simulink model "Copy_of_RL_Single_phase"  (R2020b)
settings: Solver=FixedStepDiscrete  StartTime=0.0  StopTime=Tfinal  FixedStep=SampleTime  RelTol=1e-3
InitFcn:
  | param
values from neighbouring files (symbols this model uses):
  C_DC = 1e-6    (= 1e-06)    [param.m]
  COUT = 100e-6    (= 0.0001)    [param.m]
  Cp = 1/(4*wr^2*Lp)    (= 3.29821561336e-08)    [param.m]
  Cs = 1/(4*wr^2*Ls)    (= 3.29821561336e-08)    [param.m]
  ESRA = 1e-7    (= 1e-07)    [param.m]
  ESRB = 1e-7    (= 1e-07)    [param.m]
  LCAHA = 1e-7    (= 1e-07)    [param.m]
  LCBHB = 1e-7    (= 1e-07)    [param.m]
  LHACB = 1e-7    (= 1e-07)    [param.m]
  LLoad = 2e-3    (= 0.002)    [param.m]
  Lp = 120e-6    (= 0.00012)    [param.m]
  Ls = 120e-6    (= 0.00012)    [param.m]
  LSource = 1e-7    (= 1e-07)    [param.m]
  M = 24e-6    (= 2.4e-05)    [param.m]
  phasePWM = 180    [param.m]
  RL = 12    [param.m]
  Rload = 5    [param.m]
  RSource = 1e-3    (= 0.001)    [param.m]
  SampleTime = (1/fsw)/360    (= 6.94444444444e-08)    [param.m]
  Vdc = 100    [param.m]
undefined symbols (not defined in the file or in its folder): ESLA, ESLB, Lload1, Rload1
libraries: powerlib x41, powerlib_meascontrol x2
settings Model: Creator=enes_  LastModifiedBy=enes_
settings DataIOCC: ReturnWorkspaceOutputs=off
settings DebuggingCC: ArithmeticOperatorsInVariantConditions=warning
settings SFSimCC: SimUseLocalCustomCode=off  CustomCodeUndefinedFunction=UseInterfaceOnly
settings RTWCC: RTWUseLocalCustomCode=off

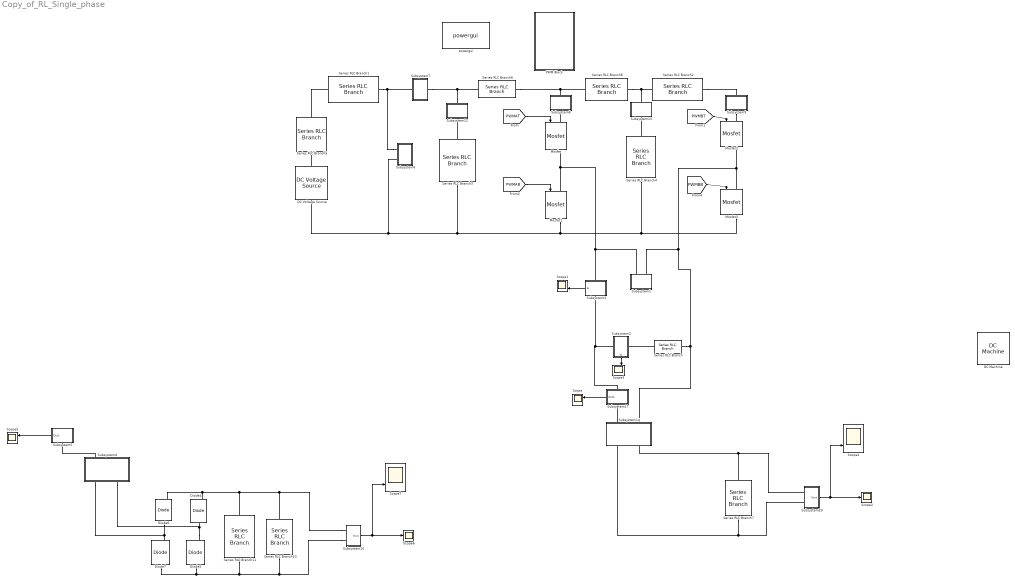
== system Copy_of_RL_Single_phase ==
  DC Machine : powerlib/Machines/DC Machine  PresetModel=No  MechanicalLoad=Torque TL  FieldType=Permanent magnet  ShowDetailedParameters=on  MeasurementBus=off  RLa="[ 0.6  0.012]"  RLf="[ 240  120]"  Laf=1.8  MachineConstant=Back-emf constant (V/rpm)  Ke=1/6  Kt=1.8  J=0.001  Bm=0  Tf=0.05  w0=0  Ifinit=1  TsPowergui=0  TsBlock=-1
  DC Voltage Source : powerlib/Electrical Sources/DC Voltage Source  Amplitude=Vdc  Measurements=None
  Diode{4..7} (4 alike) : powerlib/Power Electronics/Diode  Ron=0.001  Lon=0  Vf=0.8  IC=0  UseSnubber=0  Rs=500  Cs=250e-9  Measurements=on
  Mosfet{,1..3} (4 alike) : powerlib/Power Electronics/Mosfet  Ron=0.1  Lon=0  Rd=0.01  Vfd=0  IC=0  Rs=1e5  Cs=inf  Measurements=on
  PWM Block : Subsystem
  Scope{,1,3..5,7} (6 alike) : Scope  NumInputPorts=2
  Scope2 : Scope
  Scope6 : Scope
  Series RLC Branch : powerlib/Elements/Series RLC Branch  LConnTagsString=__new0  RConnTagsString=__new0  BranchType=RL  Resistance=Rload  Inductance=LLoad  SetiL0=off  InitialCurrent=0  Capacitance=1e-6  Setx0=off  InitialVoltage=0  Measurements=None
  Series RLC Branch1 : powerlib/Elements/Series RLC Branch  LConnTagsString=__new0  RConnTagsString=__new0  BranchType=L  Resistance=LSource  Inductance=LSource  SetiL0=off  InitialCurrent=0  Capacitance=0.01  Setx0=off  InitialVoltage=0  Measurements=None
  Series RLC Branch10 : powerlib/Elements/Series RLC Branch  LConnTagsString=__new0  RConnTagsString=__new0  BranchType=R  Resistance=RL*pi*pi/8  Inductance=Lload1  SetiL0=off  InitialCurrent=0  Capacitance=1e-6  Setx0=off  InitialVoltage=0  Measurements=None
  Series RLC Branch11 : powerlib/Elements/Series RLC Branch  LConnTagsString=__new0  RConnTagsString=__new0  BranchType=C  Resistance=ESRB  Inductance=ESLB  SetiL0=off  InitialCurrent=0  Capacitance=COUT*5  Setx0=off  InitialVoltage=0  Measurements=None
  Series RLC Branch2 : powerlib/Elements/Series RLC Branch  LConnTagsString=__new0  RConnTagsString=__new0  BranchType=L  Resistance=LSource  Inductance=LCBHB  SetiL0=off  InitialCurrent=0  Capacitance=0.01  Setx0=off  InitialVoltage=0  Measurements=None
  Series RLC Branch3 : powerlib/Elements/Series RLC Branch  LConnTagsString=__new0  RConnTagsString=__new0  BranchType=RC  Resistance=ESRA  Inductance=ESLA  SetiL0=off  InitialCurrent=0  Capacitance=C_DC  Setx0=off  InitialVoltage=0  Measurements=None
  Series RLC Branch4 : powerlib/Elements/Series RLC Branch  LConnTagsString=__new0  RConnTagsString=__new0  BranchType=RC  Resistance=ESRB  Inductance=ESLB  SetiL0=off  InitialCurrent=0  Capacitance=C_DC  Setx0=off  InitialVoltage=0  Measurements=None
  Series RLC Branch5 : powerlib/Elements/Series RLC Branch  LConnTagsString=__new0  RConnTagsString=__new0  BranchType=R  Resistance=RSource  Inductance=ESLA  SetiL0=off  InitialCurrent=0  Capacitance=0.01  Setx0=off  InitialVoltage=0  Measurements=None
  Series RLC Branch6 : powerlib/Elements/Series RLC Branch  LConnTagsString=__new0  RConnTagsString=__new0  BranchType=L  Resistance=LSource  Inductance=LCAHA  SetiL0=off  InitialCurrent=0  Capacitance=0.01  Setx0=off  InitialVoltage=0  Measurements=None
  Series RLC Branch7 : powerlib/Elements/Series RLC Branch  LConnTagsString=__new0  RConnTagsString=__new0  BranchType=R  Resistance=RL  Inductance=Lload1  SetiL0=off  InitialCurrent=0  Capacitance=1e-6  Setx0=off  InitialVoltage=0  Measurements=None
  Series RLC Branch8 : powerlib/Elements/Series RLC Branch  LConnTagsString=__new0  RConnTagsString=__new0  BranchType=L  Resistance=LSource  Inductance=LHACB  SetiL0=off  InitialCurrent=0  Capacitance=0.01  Setx0=off  InitialVoltage=0  Measurements=None
  Subsystem1 : Subsystem
  Subsystem10 : Subsystem
  Subsystem12 : Subsystem
  Subsystem13 : Subsystem
  Subsystem14 : Subsystem
      settings: PortSchema="{\"entries\":[{\"content\":{\"sides\":[{\"content\":{\"connectorIds\":[]},\"type\":\"ConnectorPlacement.EquallySpacedRectSide\",\"uuid\":\"6f1eb296-4ecd-4e86-8628-adbbf2e1adfa\"},{\"content\":{\"connectorIds\":[],\"side\":\"RIGHT\"},\"type\":\"ConnectorPlacement.EquallySpacedRectSide\",\"uuid\":\"d50ad01c-ae77-48a6-8b23-7e873a34c123\"},{\"content\":{\"connectorIds\":[\"LConn1\",\"LConn2\"],\"side\":\"TOP\"},\"type\":\"ConnectorPlacement.EquallySpacedRectSide\",\"uuid\":\"35087c95-2eb3-479b-9803-a6c51104581c\"},{\"content\":{\"connectorIds\":[\"RConn1\",\"RConn2\"],\"side\":\"BOTTOM\"},\"type\":\"ConnectorPlacement.EquallySpacedRectSide\",\"uuid\":\"95e365af-ee7d-4efb-a94a-44e2b66f7c5a\"},{\"content\":{\"connectorIds\":[],\"side\":\"HIDDEN\"},\"type\":\"ConnectorPlacement.EquallySpacedRectSide\",\"uuid\":\"7d9d40cd-59b3-4830-8a2b-338c5c07a669\"}]},\"type\":\"ConnectorPlacement.EquallySpacedConnector\",\"uuid\":\"c8ac95d6-5203-4d60-9fcb-90bc8d4d4c6c\"}],\"packageUris\":[\"http://schema.mathworks.com/mf0/Connector/R2020b\"],\"version\":\"1.0\"}"
  Subsystem17 : Subsystem
      settings: PortSchema="{\"entries\":[{\"content\":{\"sides\":[{\"content\":{\"connectorIds\":[\"LConn1\"]},\"type\":\"ConnectorPlacement.EquallySpacedRectSide\",\"uuid\":\"0f47a06b-d06e-4962-9752-b704f5a77a81\"},{\"content\":{\"connectorIds\":[\"RConn1\"],\"side\":\"RIGHT\"},\"type\":\"ConnectorPlacement.EquallySpacedRectSide\",\"uuid\":\"bcd05a72-a0a2-4c1a-8800-4f6f384a2148\"},{\"content\":{\"connectorIds\":[\"Out1\"],\"side\":\"TOP\"},\"type\":\"ConnectorPlacement.EquallySpacedRectSide\",\"uuid\":\"460eec3a-13a5-4b0a-bbe5-66a77dfd172d\"},{\"content\":{\"connectorIds\":[],\"side\":\"HIDDEN\"},\"type\":\"ConnectorPlacement.EquallySpacedRectSide\",\"uuid\":\"b74b5cc9-f01f-48bb-9528-e6a1c27da3f5\"}]},\"type\":\"ConnectorPlacement.EquallySpacedConnector\",\"uuid\":\"d4db2980-a785-4432-bb2d-fe9fde88e7eb\"}],\"packageUris\":[\"http://schema.mathworks.com/mf0/Connector/R2020b\"],\"version\":\"1.0\"}"
  Subsystem2 : Subsystem
      settings: PortSchema="{\"entries\":[{\"content\":{\"sides\":[{\"content\":{\"connectorIds\":[\"LConn1\"]},\"type\":\"ConnectorPlacement.EquallySpacedRectSide\",\"uuid\":\"0f47a06b-d06e-4962-9752-b704f5a77a81\"},{\"content\":{\"connectorIds\":[\"RConn1\"],\"side\":\"RIGHT\"},\"type\":\"ConnectorPlacement.EquallySpacedRectSide\",\"uuid\":\"bcd05a72-a0a2-4c1a-8800-4f6f384a2148\"},{\"content\":{\"connectorIds\":[\"Out1\"],\"side\":\"TOP\"},\"type\":\"ConnectorPlacement.EquallySpacedRectSide\",\"uuid\":\"460eec3a-13a5-4b0a-bbe5-66a77dfd172d\"},{\"content\":{\"connectorIds\":[],\"side\":\"HIDDEN\"},\"type\":\"ConnectorPlacement.EquallySpacedRectSide\",\"uuid\":\"b74b5cc9-f01f-48bb-9528-e6a1c27da3f5\"}]},\"type\":\"ConnectorPlacement.EquallySpacedConnector\",\"uuid\":\"d4db2980-a785-4432-bb2d-fe9fde88e7eb\"}],\"packageUris\":[\"http://schema.mathworks.com/mf0/Connector/R2020b\"],\"version\":\"1.0\"}"
  Subsystem20 : Subsystem
  Subsystem3 : Subsystem
      settings: PortSchema="{\"entries\":[{\"content\":{\"sides\":[{\"content\":{\"connectorIds\":[\"LConn1\"]},\"type\":\"ConnectorPlacement.EquallySpacedRectSide\",\"uuid\":\"0f47a06b-d06e-4962-9752-b704f5a77a81\"},{\"content\":{\"connectorIds\":[\"RConn1\"],\"side\":\"RIGHT\"},\"type\":\"ConnectorPlacement.EquallySpacedRectSide\",\"uuid\":\"bcd05a72-a0a2-4c1a-8800-4f6f384a2148\"},{\"content\":{\"connectorIds\":[\"Out1\"],\"side\":\"TOP\"},\"type\":\"ConnectorPlacement.EquallySpacedRectSide\",\"uuid\":\"460eec3a-13a5-4b0a-bbe5-66a77dfd172d\"},{\"content\":{\"connectorIds\":[],\"side\":\"HIDDEN\"},\"type\":\"ConnectorPlacement.EquallySpacedRectSide\",\"uuid\":\"b74b5cc9-f01f-48bb-9528-e6a1c27da3f5\"}]},\"type\":\"ConnectorPlacement.EquallySpacedConnector\",\"uuid\":\"d4db2980-a785-4432-bb2d-fe9fde88e7eb\"}],\"packageUris\":[\"http://schema.mathworks.com/mf0/Connector/R2020b\"],\"version\":\"1.0\"}"
  Subsystem4 : Subsystem
      settings: PortSchema="{\"entries\":[{\"content\":{\"sides\":[{\"content\":{\"connectorIds\":[]},\"type\":\"ConnectorPlacement.EquallySpacedRectSide\",\"uuid\":\"6f1eb296-4ecd-4e86-8628-adbbf2e1adfa\"},{\"content\":{\"connectorIds\":[],\"side\":\"RIGHT\"},\"type\":\"ConnectorPlacement.EquallySpacedRectSide\",\"uuid\":\"d50ad01c-ae77-48a6-8b23-7e873a34c123\"},{\"content\":{\"connectorIds\":[\"LConn1\",\"LConn2\"],\"side\":\"TOP\"},\"type\":\"ConnectorPlacement.EquallySpacedRectSide\",\"uuid\":\"35087c95-2eb3-479b-9803-a6c51104581c\"},{\"content\":{\"connectorIds\":[\"RConn1\",\"RConn2\"],\"side\":\"BOTTOM\"},\"type\":\"ConnectorPlacement.EquallySpacedRectSide\",\"uuid\":\"95e365af-ee7d-4efb-a94a-44e2b66f7c5a\"},{\"content\":{\"connectorIds\":[],\"side\":\"HIDDEN\"},\"type\":\"ConnectorPlacement.EquallySpacedRectSide\",\"uuid\":\"7d9d40cd-59b3-4830-8a2b-338c5c07a669\"}]},\"type\":\"ConnectorPlacement.EquallySpacedConnector\",\"uuid\":\"c8ac95d6-5203-4d60-9fcb-90bc8d4d4c6c\"}],\"packageUris\":[\"http://schema.mathworks.com/mf0/Connector/R2020b\"],\"version\":\"1.0\"}"
  Subsystem5 : Subsystem
      settings: PortSchema="{\"entries\":[{\"content\":{\"sides\":[{\"content\":{\"connectorIds\":[\"LConn1\"]},\"type\":\"ConnectorPlacement.EquallySpacedRectSide\",\"uuid\":\"0f47a06b-d06e-4962-9752-b704f5a77a81\"},{\"content\":{\"connectorIds\":[\"RConn1\"],\"side\":\"RIGHT\"},\"type\":\"ConnectorPlacement.EquallySpacedRectSide\",\"uuid\":\"bcd05a72-a0a2-4c1a-8800-4f6f384a2148\"},{\"content\":{\"connectorIds\":[\"Out1\"],\"side\":\"TOP\"},\"type\":\"ConnectorPlacement.EquallySpacedRectSide\",\"uuid\":\"460eec3a-13a5-4b0a-bbe5-66a77dfd172d\"},{\"content\":{\"connectorIds\":[],\"side\":\"HIDDEN\"},\"type\":\"ConnectorPlacement.EquallySpacedRectSide\",\"uuid\":\"b74b5cc9-f01f-48bb-9528-e6a1c27da3f5\"}]},\"type\":\"ConnectorPlacement.EquallySpacedConnector\",\"uuid\":\"d4db2980-a785-4432-bb2d-fe9fde88e7eb\"}],\"packageUris\":[\"http://schema.mathworks.com/mf0/Connector/R2020b\"],\"version\":\"1.0\"}"
  Subsystem6 : Subsystem
  Subsystem7 : Subsystem
  Subsystem8 : Subsystem
  Subsystem9 : Subsystem
  powergui : powerlib/powergui  Priority=1  SimulationMode=Discrete  SampleTime=SampleTime  frequency=60  Iterations=50  frequencyindice=0  Pbase=100e6  ErrMax=1e-4  UnitsV=kV  UnitsW=MW  buscounter=0  FunctionMessages=off  echomessages=off  EnableUseOfTLC=off  CurrentSourceSwitches=off  DisableSnubberDevices=off  DisableRonSwitches=off  DisableVfSwitches=off  DisplayEquations=off  AutomaticDiscreteSolvers=off  SolverType=Tustin/Backward Euler (TBE)  Interpol=off  ExternalGateDelay=off  methode=off  Ts=100  x0status=blocks  SPID=on  SwTol=0  HookPort=off  NonlinearTolerance=1e-4  nMaxIteration=100  ContinueOnMaxIteration=off  RestoreLinks=warning  ResistiveCurrentMeasurement=off  Frange=[0:2:500]  Ylog=off  Xlog=on  ShowGrid=off  save=off  variable=ZData  structure=0  ZoomFFT=off  StartTime=0.0  cycles=1  DisplayStyle=1  fundamental=60  FreqAxis=off  MaxFrequency=1000  frequencyindicesteady=1  RmsSteady=1  display=off
  wires:
  Subsystem20/1(Vout) -> Scope2/1, Scope4/2
  [PWMBT] -> Mosfet2/1
  [PWMAB] -> Mosfet1/1
  [PWMAT] -> Mosfet/1
  [PWMBB] -> Mosfet3/1
  Subsystem17/1(Out1) -> Scope/1
  Subsystem3/1(Ia) -> Scope1/2
  Subsystem2/1(Ia) -> Scope3/2
  Subsystem10/1(Vout) -> Scope6/1, Scope7/2
  Subsystem5/1(Out1) -> Scope5/1
  connections:
  Mosfet3/LConn1 -- Subsystem14/LConn2 -- Series RLC Branch/RConn1 -- Subsystem1/LConn2 -- Mosfet2/RConn1
  Subsystem2/RConn1 -- Subsystem17/RConn1 -- Subsystem3/LConn1
  Subsystem6/LConn1 -- Subsystem7/RConn1 -- Series RLC Branch1/LConn1
  Subsystem14/LConn1 -- Subsystem17/LConn1
  Series RLC Branch7/RConn1 -- Subsystem14/RConn1 -- Subsystem20/LConn2
  Series RLC Branch7/LConn1 -- Subsystem14/RConn2 -- Subsystem20/LConn1
  Series RLC Branch3/LConn1 -- Subsystem12/LConn1
  Subsystem13/RConn1 -- Series RLC Branch8/LConn1 -- Series RLC Branch2/RConn1
  Series RLC Branch4/LConn1 -- Subsystem13/LConn1
  Mosfet/LConn1 -- Subsystem8/LConn1
  Subsystem3/RConn1 -- Subsystem1/LConn1 -- Mosfet1/LConn1 -- Mosfet/RConn1
  DC Voltage Source/LConn1 -- Series RLC Branch3/RConn1 -- Mosfet1/RConn1 -- Mosfet3/RConn1 -- Series RLC Branch4/RConn1 -- Subsystem6/LConn2
  Subsystem9/LConn1 -- Mosfet2/LConn1
  DC Voltage Source/RConn1 -- Series RLC Branch5/RConn1
  Series RLC Branch5/LConn1 -- Series RLC Branch1/RConn1
  Subsystem12/RConn1 -- Subsystem7/LConn1 -- Series RLC Branch6/RConn1
  Series RLC Branch2/LConn1 -- Subsystem9/RConn1
  Series RLC Branch6/LConn1 -- Subsystem8/RConn1 -- Series RLC Branch8/RConn1
  Series RLC Branch/LConn1 -- Subsystem2/LConn1
  Diode7/RConn1 -- Diode6/LConn1 -- Subsystem4/RConn1
  Diode5/RConn1 -- Diode4/LConn1 -- Subsystem4/RConn2
  Subsystem10/LConn1 -- Series RLC Branch10/LConn1 -- Diode4/RConn1 -- Diode6/RConn1 -- Series RLC Branch11/LConn1
  Subsystem10/LConn2 -- Series RLC Branch10/RConn1 -- Diode7/LConn1 -- Diode5/LConn1 -- Series RLC Branch11/RConn1
  Subsystem4/LConn1 -- Subsystem5/LConn1

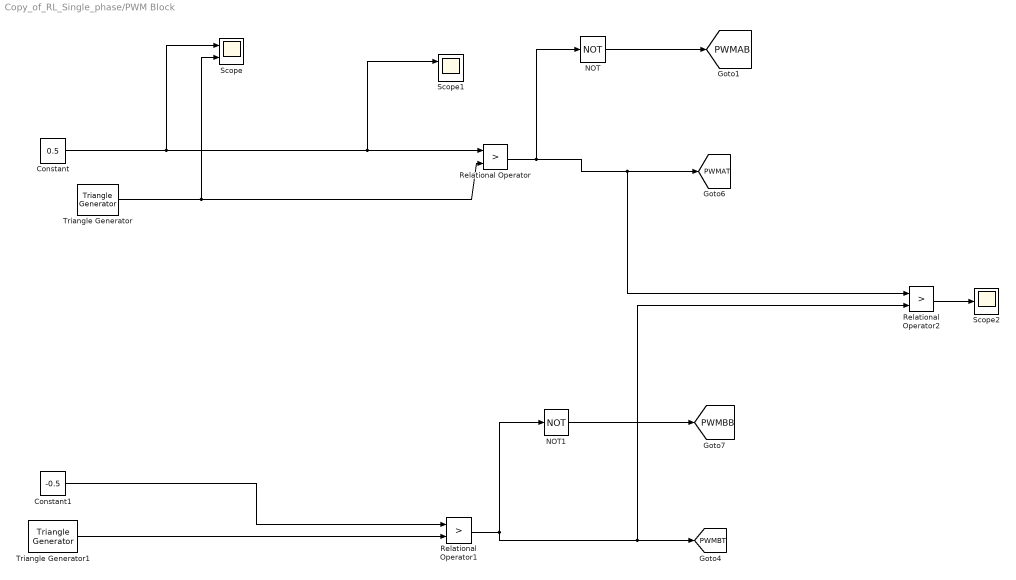
== system Copy_of_RL_Single_phase/PWM Block ==
  Constant : Constant  Value=0.5
  Constant1 : Constant  Value=-0.5
  NOT : Logic  Operator=NOT  IconShape=distinctive  AllPortsSameDT=off  OutDataTypeStr=boolean
  NOT1 : Logic  Operator=NOT  IconShape=distinctive  AllPortsSameDT=off  OutDataTypeStr=boolean
  Relational Operator : RelationalOperator  Operator=>  OutDataTypeStr=boolean  RndMeth=Simplest
  Relational Operator1 : RelationalOperator  Operator=>  OutDataTypeStr=boolean  RndMeth=Simplest
  Relational Operator2 : RelationalOperator  Operator=>  OutDataTypeStr=boolean  RndMeth=Simplest
  Scope : Scope  NumInputPorts=2
  Scope1 : Scope  NumInputPorts=2
  Scope2 : Scope
  Triangle Generator : powerlib_meascontrol/Pulse & Signal Generators/Triangle Generator  Freq=fsw  Phase=0  Ts=0
  Triangle Generator1 : powerlib_meascontrol/Pulse & Signal Generators/Triangle Generator  Freq=fsw  Phase=phasePWM  Ts=0
  tag scope: PWMAB=global, PWMAT=global, PWMBB=global, PWMBT=global
  wires:
  Triangle Generator/1 -> Relational Operator/2, Scope/2
  Constant/1 -> Scope1/1, Relational Operator/1, Scope/1
  Relational Operator/1 -> NOT/1, Relational Operator2/1, [PWMAT]
  NOT/1 -> [PWMAB]
  NOT1/1 -> [PWMBB]
  Relational Operator1/1 -> NOT1/1, Relational Operator2/2, [PWMBT]
  Triangle Generator1/1 -> Relational Operator1/2
  Constant1/1 -> Relational Operator1/1
  Relational Operator2/1 -> Scope2/1

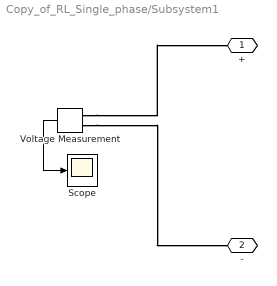
== system Copy_of_RL_Single_phase/Subsystem1 ==
  Scope : Scope
  Voltage Measurement : powerlib/Measurements/Voltage Measurement  PhasorSimulation=off  OutputType=Complex  PSBequivalent=0
  + : PMIOPort  Side=Left
  - : PMIOPort  Port=2  Side=Left
  wires:
  Voltage Measurement/1 -> Scope/1
  connections:
  Voltage Measurement/LConn1 -- +/RConn1
  Voltage Measurement/LConn2 -- -/RConn1

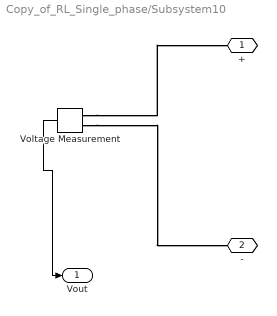
== system Copy_of_RL_Single_phase/Subsystem10 ==
  Voltage Measurement : powerlib/Measurements/Voltage Measurement  PhasorSimulation=off  OutputType=Complex  PSBequivalent=0
  + : PMIOPort  Side=Left
  - : PMIOPort  Port=2  Side=Left
  Vout : Outport  VectorParamsAs1DForOutWhenUnconnected=off
  wires:
  Voltage Measurement/1 -> Vout/1
  connections:
  Voltage Measurement/LConn1 -- +/RConn1
  Voltage Measurement/LConn2 -- -/RConn1

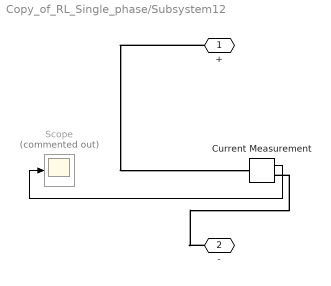
== system Copy_of_RL_Single_phase/Subsystem12 ==
  Current Measurement : powerlib/Measurements/Current Measurement  PhasorSimulation=off  OutputType=Complex  PSBequivalent=0
  Scope : Scope  Commented=on
  + : PMIOPort  Side=Right
  - : PMIOPort  Port=2  Side=Left
  wires:
  Current Measurement/1 -> Scope/1
  connections:
  +/RConn1 -- Current Measurement/LConn1
  -/RConn1 -- Current Measurement/RConn1

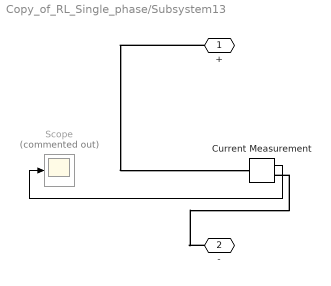
== system Copy_of_RL_Single_phase/Subsystem13 ==
  Current Measurement : powerlib/Measurements/Current Measurement  PhasorSimulation=off  OutputType=Complex  PSBequivalent=0
  Scope : Scope  Commented=on
  + : PMIOPort  Side=Right
  - : PMIOPort  Port=2  Side=Left
  wires:
  Current Measurement/1 -> Scope/1
  connections:
  +/RConn1 -- Current Measurement/LConn1
  -/RConn1 -- Current Measurement/RConn1

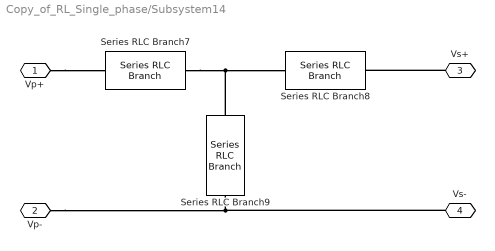
== system Copy_of_RL_Single_phase/Subsystem14 ==
  Series RLC Branch7 : powerlib/Elements/Series RLC Branch  LConnTagsString=__new0  RConnTagsString=__new0  BranchType=LC  Resistance=Rload1  Inductance=Lp-M  SetiL0=off  InitialCurrent=0  Capacitance=Cp  Setx0=off  InitialVoltage=0  Measurements=None
  Series RLC Branch8 : powerlib/Elements/Series RLC Branch  LConnTagsString=__new0  RConnTagsString=__new0  BranchType=LC  Resistance=Rload1  Inductance=Ls-M  SetiL0=off  InitialCurrent=0  Capacitance=Cs  Setx0=off  InitialVoltage=0  Measurements=None
  Series RLC Branch9 : powerlib/Elements/Series RLC Branch  LConnTagsString=__new0  RConnTagsString=__new0  BranchType=L  Resistance=Rload1  Inductance=M  SetiL0=off  InitialCurrent=0  Capacitance=Cp  Setx0=off  InitialVoltage=0  Measurements=None
  Vp+ : PMIOPort  Side=Left
  Vp- : PMIOPort  Port=2  Side=Left
  Vs+ : PMIOPort  Port=3  Side=Right
  Vs- : PMIOPort  Port=4  Side=Right
  connections:
  Series RLC Branch7/LConn1 -- Series RLC Branch9/RConn1 -- Series RLC Branch8/LConn1
  Vs+/RConn1 -- Series RLC Branch8/RConn1
  Vp+/RConn1 -- Series RLC Branch7/RConn1
  Series RLC Branch9/LConn1 -- Vs-/RConn1 -- Vp-/RConn1

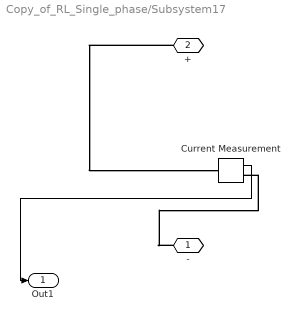
== system Copy_of_RL_Single_phase/Subsystem17 ==
  Current Measurement : powerlib/Measurements/Current Measurement  PhasorSimulation=off  OutputType=Complex  PSBequivalent=0
  - : PMIOPort  Side=Left
  + : PMIOPort  Port=2  Side=Right
  Out1 : Outport  VectorParamsAs1DForOutWhenUnconnected=off
  wires:
  Current Measurement/1 -> Out1/1
  connections:
  +/RConn1 -- Current Measurement/LConn1
  -/RConn1 -- Current Measurement/RConn1

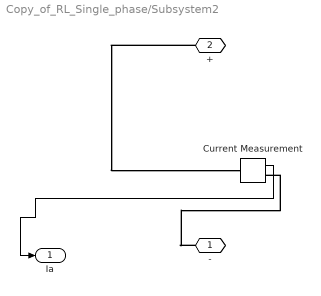
== system Copy_of_RL_Single_phase/Subsystem2 ==
  Current Measurement : powerlib/Measurements/Current Measurement  PhasorSimulation=off  OutputType=Complex  PSBequivalent=0
  - : PMIOPort  Side=Left
  + : PMIOPort  Port=2  Side=Right
  Ia : Outport  VectorParamsAs1DForOutWhenUnconnected=off
  wires:
  Current Measurement/1 -> Ia/1
  connections:
  +/RConn1 -- Current Measurement/LConn1
  -/RConn1 -- Current Measurement/RConn1

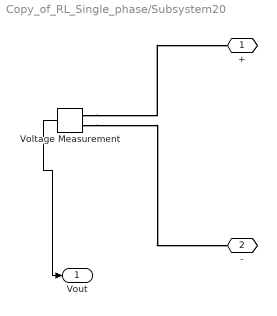
== system Copy_of_RL_Single_phase/Subsystem20 ==
  Voltage Measurement : powerlib/Measurements/Voltage Measurement  PhasorSimulation=off  OutputType=Complex  PSBequivalent=0
  + : PMIOPort  Side=Left
  - : PMIOPort  Port=2  Side=Left
  Vout : Outport  VectorParamsAs1DForOutWhenUnconnected=off
  wires:
  Voltage Measurement/1 -> Vout/1
  connections:
  Voltage Measurement/LConn1 -- +/RConn1
  Voltage Measurement/LConn2 -- -/RConn1

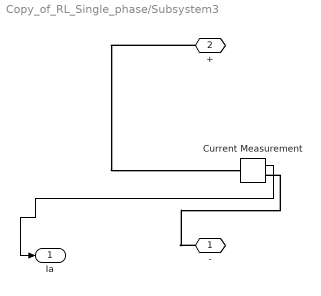
== system Copy_of_RL_Single_phase/Subsystem3 ==
  Current Measurement : powerlib/Measurements/Current Measurement  PhasorSimulation=off  OutputType=Complex  PSBequivalent=0
  - : PMIOPort  Side=Left
  + : PMIOPort  Port=2  Side=Right
  Ia : Outport  VectorParamsAs1DForOutWhenUnconnected=off
  wires:
  Current Measurement/1 -> Ia/1
  connections:
  +/RConn1 -- Current Measurement/LConn1
  -/RConn1 -- Current Measurement/RConn1

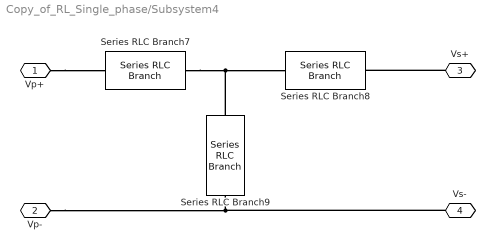
== system Copy_of_RL_Single_phase/Subsystem4 ==
  Series RLC Branch7 : powerlib/Elements/Series RLC Branch  LConnTagsString=__new0  RConnTagsString=__new0  BranchType=LC  Resistance=Rload1  Inductance=Lp-M  SetiL0=off  InitialCurrent=0  Capacitance=Cp  Setx0=off  InitialVoltage=0  Measurements=None
  Series RLC Branch8 : powerlib/Elements/Series RLC Branch  LConnTagsString=__new0  RConnTagsString=__new0  BranchType=LC  Resistance=Rload1  Inductance=Ls-M  SetiL0=off  InitialCurrent=0  Capacitance=Cs  Setx0=off  InitialVoltage=0  Measurements=None
  Series RLC Branch9 : powerlib/Elements/Series RLC Branch  LConnTagsString=__new0  RConnTagsString=__new0  BranchType=L  Resistance=Rload1  Inductance=M  SetiL0=off  InitialCurrent=0  Capacitance=Cp  Setx0=off  InitialVoltage=0  Measurements=None
  Vp+ : PMIOPort  Side=Left
  Vp- : PMIOPort  Port=2  Side=Left
  Vs+ : PMIOPort  Port=3  Side=Right
  Vs- : PMIOPort  Port=4  Side=Right
  connections:
  Series RLC Branch7/LConn1 -- Series RLC Branch9/RConn1 -- Series RLC Branch8/LConn1
  Vs+/RConn1 -- Series RLC Branch8/RConn1
  Vp+/RConn1 -- Series RLC Branch7/RConn1
  Series RLC Branch9/LConn1 -- Vs-/RConn1 -- Vp-/RConn1

== system Copy_of_RL_Single_phase/Subsystem5 ==
  Current Measurement : powerlib/Measurements/Current Measurement  PhasorSimulation=off  OutputType=Complex  PSBequivalent=0
  - : PMIOPort  Side=Left
  + : PMIOPort  Port=2  Side=Right
  Out1 : Outport  VectorParamsAs1DForOutWhenUnconnected=off
  wires:
  Current Measurement/1 -> Out1/1
  connections:
  +/RConn1 -- Current Measurement/LConn1
  -/RConn1 -- Current Measurement/RConn1

== system Copy_of_RL_Single_phase/Subsystem6 ==
  Scope : Scope
  Voltage Measurement : powerlib/Measurements/Voltage Measurement  PhasorSimulation=off  OutputType=Complex  PSBequivalent=0
  + : PMIOPort  Side=Left
  - : PMIOPort  Port=2  Side=Left
  wires:
  Voltage Measurement/1 -> Scope/1
  connections:
  Voltage Measurement/LConn1 -- +/RConn1
  Voltage Measurement/LConn2 -- -/RConn1

== system Copy_of_RL_Single_phase/Subsystem7 ==
  Current Measurement : powerlib/Measurements/Current Measurement  PhasorSimulation=off  OutputType=Complex  PSBequivalent=0
  Scope : Scope
  + : PMIOPort  Side=Right
  - : PMIOPort  Port=2  Side=Left
  wires:
  Current Measurement/1 -> Scope/1
  connections:
  +/RConn1 -- Current Measurement/LConn1
  -/RConn1 -- Current Measurement/RConn1

== system Copy_of_RL_Single_phase/Subsystem8 ==
  Current Measurement : powerlib/Measurements/Current Measurement  PhasorSimulation=off  OutputType=Complex  PSBequivalent=0
  Scope : Scope  Commented=on
  + : PMIOPort  Side=Right
  - : PMIOPort  Port=2  Side=Left
  wires:
  Current Measurement/1 -> Scope/1
  connections:
  +/RConn1 -- Current Measurement/LConn1
  -/RConn1 -- Current Measurement/RConn1

== system Copy_of_RL_Single_phase/Subsystem9 ==
  Current Measurement : powerlib/Measurements/Current Measurement  PhasorSimulation=off  OutputType=Complex  PSBequivalent=0
  Scope : Scope  Commented=on
  + : PMIOPort  Side=Right
  - : PMIOPort  Port=2  Side=Left
  wires:
  Current Measurement/1 -> Scope/1
  connections:
  +/RConn1 -- Current Measurement/LConn1
  -/RConn1 -- Current Measurement/RConn1
